simulink model "workshop5_simulink"  (R2023a)
settings: Solver=VariableStepAuto  StartTime=0.0  StopTime=25  RelTol=1e-3
values from neighbouring files (symbols this model uses):
  A = [0, 1; -k/m, -b/m]    [workshop5.m]
  B = [0; 1/m]    [workshop5.m]
  C = [1, 0]    [workshop5.m]
settings Model: Creator=seanmcgowan  LastModifiedBy=seanmcgowan

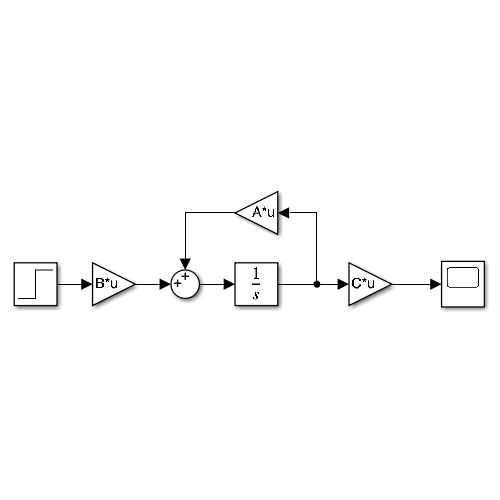
[thumbnail: Simulink's stored preview of the top-level diagram]
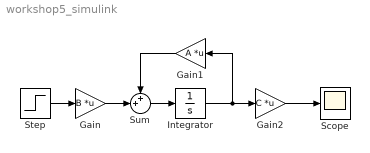
== system workshop5_simulink ==
  Gain : Gain  Gain=B  Multiplication=Matrix(K*u)
  Gain1 : Gain  Gain=A  Multiplication=Matrix(K*u)
  Gain2 : Gain  Gain=C  Multiplication=Matrix(K*u)
  Integrator : Integrator
  Scope : Scope
  Step : Step  Time=0  SampleTime=0
  Sum : Sum  Inputs=++|
  wires:
  Gain/1 -> Sum/2
  Sum/1 -> Integrator/1
  Integrator/1 -> Gain1/1, Gain2/1
  Gain1/1 -> Sum/1
  Step/1 -> Gain/1
  Gain2/1 -> Scope/1
